simulink model "Simscape_Benchmark_SIM1"  (R2021a)
settings: Solver=ode45  StartTime=0.0  StopTime=PHASE.Ttotal  FixedStep=Benchmark.Sim.Tint  RelTol=1e-5  AbsTol=1e-6
undefined symbols (not defined in the file): Actuators, Analysis, antisym, Benchmark, Bus, Disturbance, FSM, IntialCond, ISOL, K_Coarse_disc_t, Kslew_opt_disc_zoh, Model, MPS, PAYLOAD, PHASE, PMA, RWIsol, RWS, SA, Sensors, Slew, slosh, thr, X, Y, Z
libraries: sm_lib x215, nesl_utility x148, simulink x65, cstblocks x36, sharedtransform x4, vrlib x3, RCTblocks x1
(part 9 of 9)

== system Simscape_Benchmark_SIM1/Dynamical system/WEMS + Reaction wheels/RW saturation and friction model/Saturations + friction model + friction spikes/Spike generation RW2 ==
  note: The condition above triggers the calculation of the spike level and the repetition time.
      | While the time_counter < Rep_time the trigger is not activated. As soon as the condition is met. The logical operator {>} activates the trigger_spike subsystem and resets the counter.
  note: maybe there's a better way to round up numbers to a certain decimal in simulink but that works fine for now
  note: The function counts how many times the {>} is activated. The output values is also used in the selection of the first repetition time since this is not initialized with trigger_spike.
  note: This part is done to avoid having a first spike always at t=t_duration of spike (which is 20 sec in this case)...so we have a trigger that for the first time (when the subsystem that computes the spike repetition time has still not been triggered) choose the time of the first initial spike.... the other time will be the t_duration that sums yp with the spike repetition time
  Constant16 : Constant  Value=RWS.spike.duration
  Constant17 : Constant  Value=0  SampleTime=Model.ACS_sampling.Ts
  Constant18 : Constant  Value=RWS.spike.repetition.w2_Initialization  SampleTime=Inf
  Constant4 : Constant  Value=0  SampleTime=Model.ACS_sampling.Ts
  Couter with reset function given by a condition : Subsystem
  Gain4 : Gain  Gain=10
  Gain5 : Gain  Gain=1/10
  Memory{12..15} (4 alike) : Memory
  Relational Operator3 : RelationalOperator  Operator=>  OutDataTypeStr=boolean  RndMeth=Simplest
  Round2 : Rounding  Operator=round
  Scope{5,15,20..22} (5 alike) : Scope
  Scope23 : Scope  NumInputPorts=3
  Set_spike_duration : MATLAB Function  TreatAsAtomicUnit=on
  Sum2 : Sum  Inputs=|++
  Sum8 : Sum  Inputs=|++
  Switch3 : Switch  Criteria=u2 > Threshold  Threshold=RWS.spike.duration/Model.ACS_sampling.Ts
  Switch7 : Switch  Criteria=u2 > Threshold  Threshold=1
  Trigger_spike : Subsystem  TreatAsAtomicUnit=on
  Triggered_spikes_counter : Subsystem  TreatAsAtomicUnit=on
  Out1 : Outport
  wires:
  Constant16/1 -> Switch7/1
  Sum8/1 -> Relational Operator3/2, Scope20/1
  Gain5/1 -> Switch7/3
  Set_spike_duration/1(y) -> Switch3/2, Memory15/1
  Relational Operator3/1 -> Scope23/2, Triggered_spikes_counter/Trigger, Couter with reset function given by a condition/1(In1), Trigger_spike/Trigger
  Constant18/1 -> Gain4/1
  Sum2/1 -> Set_spike_duration/3(counter)
  Constant4/1 -> Sum2/1
  Round2/1 -> Gain5/1
  Memory12/1 -> Set_spike_duration/2(uk_1)
  Memory13/1 -> Sum8/1
  Trigger_spike/1(Spike_level) -> Set_spike_duration/1(uk), Switch3/3, Memory12/1, Scope5/1, Scope23/1
  Memory14/1 -> Sum8/2
  Trigger_spike/2(Rep_time) -> Memory13/1
  Switch3/1 -> Out1/1, Scope21/1  "Spike(t)"
  Constant17/1 -> Switch3/1
  Memory15/1 -> Sum2/2
  Triggered_spikes_counter/1(Out1) -> Scope15/1, Switch7/2
  Gain4/1 -> Round2/1
  Couter with reset function given by a condition/1(Time_counter) -> Relational Operator3/1, Scope23/3
  Switch7/1 -> Scope22/1, Memory14/1

== system Simscape_Benchmark_SIM1/Dynamical system/WEMS + Reaction wheels/RW saturation and friction model/Saturations + friction model + friction spikes/Spike generation RW3 ==
  note: The condition above triggers the calculation of the spike level and the repetition time.
      | While the time_counter < Rep_time the trigger is not activated. As soon as the condition is met. The logical operator {>} activates the trigger_spike subsystem and resets the counter.
  note: maybe there's a better way to round up numbers to a certain decimal in simulink but that works fine for now
  note: The function counts how many times the {>} is activated. The output values is also used in the selection of the first repetition time since this is not initialized with trigger_spike.
  note: This part is done to avoid having a first spike always at t=t_duration of spike (which is 20 sec in this case)...so we have a trigger that for the first time (when the subsystem that computes the spike repetition time has still not been triggered) choose the time of the first initial spike.... the other time will be the t_duration that sums yp with the spike repetition time
  Constant16 : Constant  Value=RWS.spike.duration
  Constant17 : Constant  Value=0  SampleTime=Model.ACS_sampling.Ts
  Constant18 : Constant  Value=RWS.spike.repetition.w3_Initialization  SampleTime=Inf
  Constant4 : Constant  Value=0  SampleTime=Model.ACS_sampling.Ts
  Couter with reset function given by a condition : Subsystem
  Gain4 : Gain  Gain=10
  Gain5 : Gain  Gain=1/10
  Memory{12..15} (4 alike) : Memory
  Relational Operator3 : RelationalOperator  Operator=>  OutDataTypeStr=boolean  RndMeth=Simplest
  Round2 : Rounding  Operator=round
  Scope{5,15,20..22} (5 alike) : Scope
  Scope23 : Scope  NumInputPorts=3
  Set_spike_duration : MATLAB Function  TreatAsAtomicUnit=on
  Sum2 : Sum  Inputs=|++
  Sum8 : Sum  Inputs=|++
  Switch3 : Switch  Criteria=u2 > Threshold  Threshold=RWS.spike.duration/Model.ACS_sampling.Ts
  Switch7 : Switch  Criteria=u2 > Threshold  Threshold=1
  Trigger_spike : Subsystem  TreatAsAtomicUnit=on
  Triggered_spikes_counter : Subsystem  TreatAsAtomicUnit=on
  Out1 : Outport
  wires:
  Constant16/1 -> Switch7/1
  Sum8/1 -> Relational Operator3/2, Scope20/1
  Gain5/1 -> Switch7/3
  Set_spike_duration/1(y) -> Switch3/2, Memory15/1
  Relational Operator3/1 -> Scope23/2, Triggered_spikes_counter/Trigger, Couter with reset function given by a condition/1(In1), Trigger_spike/Trigger
  Constant18/1 -> Gain4/1
  Sum2/1 -> Set_spike_duration/3(counter)
  Constant4/1 -> Sum2/1
  Round2/1 -> Gain5/1
  Memory12/1 -> Set_spike_duration/2(uk_1)
  Memory13/1 -> Sum8/1
  Trigger_spike/1(Spike_level) -> Set_spike_duration/1(uk), Switch3/3, Memory12/1, Scope5/1, Scope23/1
  Memory14/1 -> Sum8/2
  Trigger_spike/2(Rep_time) -> Memory13/1
  Switch3/1 -> Out1/1, Scope21/1  "Spike(t)"
  Constant17/1 -> Switch3/1
  Memory15/1 -> Sum2/2
  Triggered_spikes_counter/1(Out1) -> Scope15/1, Switch7/2
  Gain4/1 -> Round2/1
  Couter with reset function given by a condition/1(Time_counter) -> Relational Operator3/1, Scope23/3
  Switch7/1 -> Scope22/1, Memory14/1

== system Simscape_Benchmark_SIM1/Dynamical system/WEMS + Reaction wheels/RW saturation and friction model/Saturations + friction model + friction spikes/Spike generation RW4 ==
  note: The condition above triggers the calculation of the spike level and the repetition time.
      | While the time_counter < Rep_time the trigger is not activated. As soon as the condition is met. The logical operator {>} activates the trigger_spike subsystem and resets the counter.
  note: maybe there's a better way to round up numbers to a certain decimal in simulink but that works fine for now
  note: The function counts how many times the {>} is activated. The output values is also used in the selection of the first repetition time since this is not initialized with trigger_spike.
  note: This part is done to avoid having a first spike always at t=t_duration of spike (which is 20 sec in this case)...so we have a trigger that for the first time (when the subsystem that computes the spike repetition time has still not been triggered) choose the time of the first initial spike.... the other time will be the t_duration that sums yp with the spike repetition time
  Constant16 : Constant  Value=RWS.spike.duration
  Constant17 : Constant  Value=0  SampleTime=Model.ACS_sampling.Ts
  Constant18 : Constant  Value=RWS.spike.repetition.w4_Initialization  SampleTime=Inf
  Constant4 : Constant  Value=0  SampleTime=Model.ACS_sampling.Ts
  Couter with reset function given by a condition : Subsystem
  Gain4 : Gain  Gain=10
  Gain5 : Gain  Gain=1/10
  Memory{12..15} (4 alike) : Memory
  Relational Operator3 : RelationalOperator  Operator=>  OutDataTypeStr=boolean  RndMeth=Simplest
  Round2 : Rounding  Operator=round
  Scope{5,15,20..22} (5 alike) : Scope
  Scope23 : Scope  NumInputPorts=3
  Set_spike_duration : MATLAB Function  TreatAsAtomicUnit=on
  Sum2 : Sum  Inputs=|++
  Sum8 : Sum  Inputs=|++
  Switch3 : Switch  Criteria=u2 > Threshold  Threshold=RWS.spike.duration/Model.ACS_sampling.Ts
  Switch7 : Switch  Criteria=u2 > Threshold  Threshold=1
  Trigger_spike : Subsystem  TreatAsAtomicUnit=on
  Triggered_spikes_counter : Subsystem  TreatAsAtomicUnit=on
  Out1 : Outport
  wires:
  Constant16/1 -> Switch7/1
  Sum8/1 -> Relational Operator3/2, Scope20/1
  Gain5/1 -> Switch7/3
  Set_spike_duration/1(y) -> Switch3/2, Memory15/1
  Relational Operator3/1 -> Scope23/2, Triggered_spikes_counter/Trigger, Couter with reset function given by a condition/1(In1), Trigger_spike/Trigger
  Constant18/1 -> Gain4/1
  Sum2/1 -> Set_spike_duration/3(counter)
  Constant4/1 -> Sum2/1
  Round2/1 -> Gain5/1
  Memory12/1 -> Set_spike_duration/2(uk_1)
  Memory13/1 -> Sum8/1
  Trigger_spike/1(Spike_level) -> Set_spike_duration/1(uk), Switch3/3, Memory12/1, Scope5/1, Scope23/1
  Memory14/1 -> Sum8/2
  Trigger_spike/2(Rep_time) -> Memory13/1
  Switch3/1 -> Out1/1, Scope21/1  "Spike(t)"
  Constant17/1 -> Switch3/1
  Memory15/1 -> Sum2/2
  Triggered_spikes_counter/1(Out1) -> Scope15/1, Switch7/2
  Gain4/1 -> Round2/1
  Couter with reset function given by a condition/1(Time_counter) -> Relational Operator3/1, Scope23/3
  Switch7/1 -> Scope22/1, Memory14/1

== system Simscape_Benchmark_SIM1/Dynamical system/WEMS + Reaction wheels/RW saturation and friction model/Saturations +  friction model/RW friction model/Friction model (torque) ==
  rw_speed (rad/s) : Inport
  motor cmd trq (Nm) : Inport  Port=2
  Computation of the sign of rw_speed : Subsystem
  Friction torque calculation : Subsystem
  Sum : Sum  Inputs=+++  SaturateOnIntegerOverflow=on
  Sum1 : Sum  SaturateOnIntegerOverflow=on
  Torque_total : Outport  VectorParamsAs1DForOutWhenUnconnected=off
  Torque_friction : Outport  Port=2  VectorParamsAs1DForOutWhenUnconnected=off
  wires:
  rw_speed (rad/s)/1 -> Computation of the sign of rw_speed/1(rw_speed), Friction torque calculation/1(rw_speed)
  Computation of the sign of rw_speed/1(sign_rw_speed) -> Friction torque calculation/2(sign_rw_speed)
  Friction torque calculation/2(Torque_stiction) -> Sum/2
  Friction torque calculation/1(Torque_Coulomb) -> Sum/1
  Sum1/1 -> Torque_total/1
  Friction torque calculation/3(Torque_viscous) -> Sum/3
  Sum/1 -> Torque_friction/1, Sum1/1
  motor cmd trq (Nm)/1 -> Computation of the sign of rw_speed/2(Torque_motor), Sum1/2

== system Simscape_Benchmark_SIM1/Dynamical system/WEMS + Reaction wheels/RW saturation and friction model/Saturations + friction model + friction spikes/RW friction model/Friction model (torque)1 ==
  rw_speed (rad/s) : Inport
  motor cmd trq (Nm) : Inport  Port=2
  Computation of the sign of rw_speed : Subsystem
  Friction torque calculation : Subsystem
  Sum : Sum  Inputs=+++  SaturateOnIntegerOverflow=on
  Sum1 : Sum  SaturateOnIntegerOverflow=on
  Torque_total : Outport  VectorParamsAs1DForOutWhenUnconnected=off
  Torque_friction : Outport  Port=2  VectorParamsAs1DForOutWhenUnconnected=off
  sign_omega : Outport  Port=3
  wires:
  rw_speed (rad/s)/1 -> Computation of the sign of rw_speed/1(rw_speed), Friction torque calculation/1(rw_speed)
  Friction torque calculation/2(Torque_stiction) -> Sum/2
  Friction torque calculation/1(Torque_Coulomb) -> Sum/1
  Sum1/1 -> Torque_total/1
  Friction torque calculation/3(Torque_viscous) -> Sum/3
  Sum/1 -> Torque_friction/1, Sum1/1
  motor cmd trq (Nm)/1 -> Computation of the sign of rw_speed/2(Torque_motor), Sum1/2
  Computation of the sign of rw_speed/1(sign_rw_speed) -> sign_omega/1, Friction torque calculation/2(sign_rw_speed)

== system Simscape_Benchmark_SIM1/Dynamical system/WEMS + Reaction wheels/RW saturation and friction model/Saturations + friction model + friction spikes/Spike generation RW1/Couter with reset function given by a condition ==
  note: When the IF condition of the switch is met the counter gets reset at zero
  In1 : Inport
  Constant10 : Constant  SampleTime=Model.ACS_sampling.Ts
  Constant12 : Constant  Value=0  SampleTime=Model.ACS_sampling.Ts
  Delay : Delay  DelayLength=1  SampleTime=Model.ACS_sampling.Ts
  Memory17 : Memory  InheritSampleTime=on
  Scope18 : Scope
  Sum7 : Sum  Inputs=|++
  Switch6 : Switch  Criteria=u2 > Threshold
  Ts : Gain  Gain=Model.ACS_sampling.Ts
  Time_counter : Outport
  wires:
  Sum7/1 -> Switch6/3
  Constant10/1 -> Ts/1
  Ts/1 -> Sum7/1
  Constant12/1 -> Switch6/1
  Switch6/1 -> Delay/1, Time_counter/1, Scope18/1
  In1/1 -> Memory17/1
  Memory17/1 -> Switch6/2
  Delay/1 -> Sum7/2

== system Simscape_Benchmark_SIM1/Dynamical system/WEMS + Reaction wheels/RW saturation and friction model/Saturations + friction model + friction spikes/Spike generation RW1/Trigger_spike ==
  note: way to round up at first decimal term
  Trigger : TriggerPort  VariantControl=Variant
  Constant : Constant  Value=RWS.spike.level.bias
  Constant1 : Constant  Value=RWS.spike.repetition.bias
  Gain : Gain  Gain=10
  Gain1 : Gain  Gain=1/10
  Gain2 : Gain  Gain=RWS.spike.level.scaling
  Gain3 : Gain  Gain=1/RWS.spike.level.rate
  Gain4 : Gain  Gain=1/RWS.spike.repetition.rate
  Gain5 : Gain  Gain=RWS.spike.mN2N
  Log : Math  Operator=log  SaturateOnIntegerOverflow=on
  Log2 : Math  Operator=log  SaturateOnIntegerOverflow=on
  Product : Product
  Round : Rounding  Operator=round
  Scope : Scope
  Sum : Sum  Inputs=-+
  Sum1 : Sum  Inputs=-+
  Uniform Random Number : UniformRandomNumber  Minimum=0  Seed=RWS.spike.w1seed(1)
  Uniform Random Number1 : UniformRandomNumber  Minimum=0  Seed=RWS.spike.w1seed(2)
  Uniform Random Number2 : UniformRandomNumber  Minimum=0  Seed=RWS.spike.w1seed(3)
  Spike_level : Outport
  Rep_time : Outport  Port=2
  wires:
  Gain2/1 -> Spike_level/1
  Sum1/1 -> Gain/1
  Gain1/1 -> Rep_time/1
  Gain/1 -> Round/1
  Round/1 -> Gain1/1
  Uniform Random Number/1 -> Product/1
  Uniform Random Number1/1 -> Product/2
  Constant/1 -> Sum/2
  Gain5/1 -> Gain2/1
  Product/1 -> Log/1
  Log/1 -> Gain3/1
  Gain3/1 -> Scope/1, Sum/1
  Gain4/1 -> Sum1/1
  Uniform Random Number2/1 -> Log2/1
  Constant1/1 -> Sum1/2
  Log2/1 -> Gain4/1
  Sum/1 -> Gain5/1

== system Simscape_Benchmark_SIM1/Dynamical system/WEMS + Reaction wheels/RW saturation and friction model/Saturations + friction model + friction spikes/Spike generation RW1/Triggered_spikes_counter ==
  Trigger : TriggerPort  VariantControl=Variant
  Constant12 : Constant  Value=0
  Increment Stored Integer2 : simulink/Additional Math & Discrete/Additional Math: Increment - Decrement/Increment Stored Integer
  Sum8 : Sum
  Unit Delay1 : UnitDelay  SampleTime=-1  HasFrameUpgradeWarning=on
  Out1 : Outport
  wires:
  Constant12/1 -> Sum8/2
  Sum8/1 -> Increment Stored Integer2/1
  Unit Delay1/1 -> Sum8/1
  Increment Stored Integer2/1 -> Unit Delay1/1, Out1/1

== system Simscape_Benchmark_SIM1/Dynamical system/WEMS + Reaction wheels/RW saturation and friction model/Saturations + friction model + friction spikes/Spike generation RW2/Couter with reset function given by a condition ==
  note: When the IF condition of the switch is met the counter gets reset at zero
  In1 : Inport
  Constant10 : Constant  SampleTime=Model.ACS_sampling.Ts
  Constant12 : Constant  Value=0  SampleTime=Model.ACS_sampling.Ts
  Delay : Delay  DelayLength=1  SampleTime=Model.ACS_sampling.Ts
  Memory17 : Memory
  Scope18 : Scope
  Sum7 : Sum  Inputs=|++
  Switch6 : Switch  Criteria=u2 > Threshold
  Ts : Gain  Gain=Model.ACS_sampling.Ts
  Time_counter : Outport
  wires:
  Sum7/1 -> Switch6/3
  Constant10/1 -> Ts/1
  Ts/1 -> Sum7/1
  Constant12/1 -> Switch6/1
  Switch6/1 -> Delay/1, Time_counter/1, Scope18/1
  In1/1 -> Memory17/1
  Memory17/1 -> Switch6/2
  Delay/1 -> Sum7/2

== system Simscape_Benchmark_SIM1/Dynamical system/WEMS + Reaction wheels/RW saturation and friction model/Saturations + friction model + friction spikes/Spike generation RW2/Trigger_spike ==
  note: way to round up at first decimal term
  Trigger : TriggerPort  VariantControl=Variant
  Constant : Constant  Value=RWS.spike.level.bias
  Constant1 : Constant  Value=RWS.spike.repetition.bias
  Gain : Gain  Gain=10
  Gain1 : Gain  Gain=1/10
  Gain2 : Gain  Gain=RWS.spike.level.scaling
  Gain3 : Gain  Gain=1/RWS.spike.level.rate
  Gain4 : Gain  Gain=1/RWS.spike.repetition.rate
  Gain5 : Gain  Gain=RWS.spike.mN2N
  Log : Math  Operator=log  SaturateOnIntegerOverflow=on
  Log2 : Math  Operator=log  SaturateOnIntegerOverflow=on
  Product : Product
  Round : Rounding  Operator=round
  Scope : Scope
  Sum : Sum  Inputs=-+
  Sum1 : Sum  Inputs=-+
  Uniform Random Number : UniformRandomNumber  Minimum=0  Seed=RWS.spike.w2seed(1)
  Uniform Random Number1 : UniformRandomNumber  Minimum=0  Seed=RWS.spike.w2seed(2)
  Uniform Random Number2 : UniformRandomNumber  Minimum=0  Seed=RWS.spike.w2seed(3)
  Spike_level : Outport
  Rep_time : Outport  Port=2
  wires:
  Gain2/1 -> Spike_level/1
  Sum1/1 -> Gain/1
  Gain1/1 -> Rep_time/1
  Gain/1 -> Round/1
  Round/1 -> Gain1/1
  Uniform Random Number/1 -> Product/1
  Uniform Random Number1/1 -> Product/2
  Constant/1 -> Sum/2
  Gain5/1 -> Gain2/1
  Product/1 -> Log/1
  Log/1 -> Gain3/1
  Gain3/1 -> Scope/1, Sum/1
  Gain4/1 -> Sum1/1
  Uniform Random Number2/1 -> Log2/1
  Constant1/1 -> Sum1/2
  Log2/1 -> Gain4/1
  Sum/1 -> Gain5/1

== system Simscape_Benchmark_SIM1/Dynamical system/WEMS + Reaction wheels/RW saturation and friction model/Saturations + friction model + friction spikes/Spike generation RW2/Triggered_spikes_counter ==
  Trigger : TriggerPort  VariantControl=Variant
  Constant12 : Constant  Value=0
  Increment Stored Integer2 : simulink/Additional Math & Discrete/Additional Math: Increment - Decrement/Increment Stored Integer
  Sum8 : Sum
  Unit Delay1 : UnitDelay  SampleTime=-1  HasFrameUpgradeWarning=on
  Out1 : Outport
  wires:
  Constant12/1 -> Sum8/2
  Sum8/1 -> Increment Stored Integer2/1
  Unit Delay1/1 -> Sum8/1
  Increment Stored Integer2/1 -> Unit Delay1/1, Out1/1

== system Simscape_Benchmark_SIM1/Dynamical system/WEMS + Reaction wheels/RW saturation and friction model/Saturations + friction model + friction spikes/Spike generation RW3/Couter with reset function given by a condition ==
  note: When the IF condition of the switch is met the counter gets reset at zero
  In1 : Inport
  Constant10 : Constant  SampleTime=Model.ACS_sampling.Ts
  Constant12 : Constant  Value=0  SampleTime=Model.ACS_sampling.Ts
  Delay : Delay  DelayLength=1  SampleTime=Model.ACS_sampling.Ts
  Memory17 : Memory
  Scope18 : Scope
  Sum7 : Sum  Inputs=|++
  Switch6 : Switch  Criteria=u2 > Threshold
  Ts : Gain  Gain=Model.ACS_sampling.Ts
  Time_counter : Outport
  wires:
  Sum7/1 -> Switch6/3
  Constant10/1 -> Ts/1
  Ts/1 -> Sum7/1
  Constant12/1 -> Switch6/1
  Switch6/1 -> Delay/1, Time_counter/1, Scope18/1
  In1/1 -> Memory17/1
  Memory17/1 -> Switch6/2
  Delay/1 -> Sum7/2

== system Simscape_Benchmark_SIM1/Dynamical system/WEMS + Reaction wheels/RW saturation and friction model/Saturations + friction model + friction spikes/Spike generation RW3/Trigger_spike ==
  note: way to round up at first decimal term
  Trigger : TriggerPort  VariantControl=Variant
  Constant : Constant  Value=RWS.spike.level.bias
  Constant1 : Constant  Value=RWS.spike.repetition.bias
  Gain : Gain  Gain=10
  Gain1 : Gain  Gain=1/10
  Gain2 : Gain  Gain=RWS.spike.level.scaling
  Gain3 : Gain  Gain=1/RWS.spike.level.rate
  Gain4 : Gain  Gain=1/RWS.spike.repetition.rate
  Gain5 : Gain  Gain=RWS.spike.mN2N
  Log : Math  Operator=log  SaturateOnIntegerOverflow=on
  Log2 : Math  Operator=log  SaturateOnIntegerOverflow=on
  Product : Product
  Round : Rounding  Operator=round
  Scope : Scope
  Sum : Sum  Inputs=-+
  Sum1 : Sum  Inputs=-+
  Uniform Random Number : UniformRandomNumber  Minimum=0  Seed=RWS.spike.w3seed(1)
  Uniform Random Number1 : UniformRandomNumber  Minimum=0  Seed=RWS.spike.w3seed(2)
  Uniform Random Number2 : UniformRandomNumber  Minimum=0  Seed=RWS.spike.w3seed(3)
  Spike_level : Outport
  Rep_time : Outport  Port=2
  wires:
  Gain2/1 -> Spike_level/1
  Sum1/1 -> Gain/1
  Gain1/1 -> Rep_time/1
  Gain/1 -> Round/1
  Round/1 -> Gain1/1
  Uniform Random Number/1 -> Product/1
  Uniform Random Number1/1 -> Product/2
  Constant/1 -> Sum/2
  Gain5/1 -> Gain2/1
  Product/1 -> Log/1
  Log/1 -> Gain3/1
  Gain3/1 -> Scope/1, Sum/1
  Gain4/1 -> Sum1/1
  Uniform Random Number2/1 -> Log2/1
  Constant1/1 -> Sum1/2
  Log2/1 -> Gain4/1
  Sum/1 -> Gain5/1

== system Simscape_Benchmark_SIM1/Dynamical system/WEMS + Reaction wheels/RW saturation and friction model/Saturations + friction model + friction spikes/Spike generation RW3/Triggered_spikes_counter ==
  Trigger : TriggerPort  VariantControl=Variant
  Constant12 : Constant  Value=0
  Increment Stored Integer2 : simulink/Additional Math & Discrete/Additional Math: Increment - Decrement/Increment Stored Integer
  Sum8 : Sum
  Unit Delay1 : UnitDelay  SampleTime=-1  HasFrameUpgradeWarning=on
  Out1 : Outport
  wires:
  Constant12/1 -> Sum8/2
  Sum8/1 -> Increment Stored Integer2/1
  Unit Delay1/1 -> Sum8/1
  Increment Stored Integer2/1 -> Unit Delay1/1, Out1/1

== system Simscape_Benchmark_SIM1/Dynamical system/WEMS + Reaction wheels/RW saturation and friction model/Saturations + friction model + friction spikes/Spike generation RW4/Couter with reset function given by a condition ==
  note: When the IF condition of the switch is met the counter gets reset at zero
  In1 : Inport
  Constant10 : Constant  SampleTime=Model.ACS_sampling.Ts
  Constant12 : Constant  Value=0  SampleTime=Model.ACS_sampling.Ts
  Delay : Delay  DelayLength=1  SampleTime=Model.ACS_sampling.Ts
  Memory17 : Memory
  Scope18 : Scope
  Sum7 : Sum  Inputs=|++
  Switch6 : Switch  Criteria=u2 > Threshold
  Ts : Gain  Gain=Model.ACS_sampling.Ts
  Time_counter : Outport
  wires:
  Sum7/1 -> Switch6/3
  Constant10/1 -> Ts/1
  Ts/1 -> Sum7/1
  Constant12/1 -> Switch6/1
  Switch6/1 -> Delay/1, Time_counter/1, Scope18/1
  In1/1 -> Memory17/1
  Memory17/1 -> Switch6/2
  Delay/1 -> Sum7/2

== system Simscape_Benchmark_SIM1/Dynamical system/WEMS + Reaction wheels/RW saturation and friction model/Saturations + friction model + friction spikes/Spike generation RW4/Trigger_spike ==
  note: way to round up at first decimal term
  Trigger : TriggerPort  VariantControl=Variant
  Constant : Constant  Value=RWS.spike.level.bias
  Constant1 : Constant  Value=RWS.spike.repetition.bias
  Gain : Gain  Gain=10
  Gain1 : Gain  Gain=1/10
  Gain2 : Gain  Gain=RWS.spike.level.scaling
  Gain3 : Gain  Gain=1/RWS.spike.level.rate
  Gain4 : Gain  Gain=1/RWS.spike.repetition.rate
  Gain5 : Gain  Gain=RWS.spike.mN2N
  Log : Math  Operator=log  SaturateOnIntegerOverflow=on
  Log2 : Math  Operator=log  SaturateOnIntegerOverflow=on
  Product : Product
  Round : Rounding  Operator=round
  Scope : Scope
  Sum : Sum  Inputs=-+
  Sum1 : Sum  Inputs=-+
  Uniform Random Number : UniformRandomNumber  Minimum=0  Seed=RWS.spike.w4seed(1)
  Uniform Random Number1 : UniformRandomNumber  Minimum=0  Seed=RWS.spike.w4seed(2)
  Uniform Random Number2 : UniformRandomNumber  Minimum=0  Seed=RWS.spike.w4seed(3)
  Spike_level : Outport
  Rep_time : Outport  Port=2
  wires:
  Gain2/1 -> Spike_level/1
  Sum1/1 -> Gain/1
  Gain1/1 -> Rep_time/1
  Gain/1 -> Round/1
  Round/1 -> Gain1/1
  Uniform Random Number/1 -> Product/1
  Uniform Random Number1/1 -> Product/2
  Constant/1 -> Sum/2
  Gain5/1 -> Gain2/1
  Product/1 -> Log/1
  Log/1 -> Gain3/1
  Gain3/1 -> Scope/1, Sum/1
  Gain4/1 -> Sum1/1
  Uniform Random Number2/1 -> Log2/1
  Constant1/1 -> Sum1/2
  Log2/1 -> Gain4/1
  Sum/1 -> Gain5/1

== system Simscape_Benchmark_SIM1/Dynamical system/WEMS + Reaction wheels/RW saturation and friction model/Saturations + friction model + friction spikes/Spike generation RW4/Triggered_spikes_counter ==
  Trigger : TriggerPort  VariantControl=Variant
  Constant12 : Constant  Value=0
  Increment Stored Integer2 : simulink/Additional Math & Discrete/Additional Math: Increment - Decrement/Increment Stored Integer
  Sum8 : Sum
  Unit Delay1 : UnitDelay  SampleTime=-1  HasFrameUpgradeWarning=on
  Out1 : Outport
  wires:
  Constant12/1 -> Sum8/2
  Sum8/1 -> Increment Stored Integer2/1
  Unit Delay1/1 -> Sum8/1
  Increment Stored Integer2/1 -> Unit Delay1/1, Out1/1

== system Simscape_Benchmark_SIM1/Dynamical system/WEMS + Reaction wheels/RW saturation and friction model/Saturations +  friction model/RW friction model/Friction model (torque)/Computation of the sign of rw_speed ==
  note: IF [rw_speed| <= eps AND |Torque_motor|>eps then:
      | sign( rw_speed )=Torque_motor/|Torque_motor|
      |
      | IF [ rw_speed | <= eps and | Torque_motor |<= eps then sign( rw_speed )=0 so zero friction
  note: IF |rw_speed|>eps (tolerance given in input):
      | Then sign(rw_speed)=rw_speed/|rw_speed|
  rw_speed : Inport
  Torque_motor : Inport  Port=2
  Abs2 : Abs  SaturateOnIntegerOverflow=on
  Abs3 : Abs  SaturateOnIntegerOverflow=on
  Add : Sum  Inputs=+++
  Constant{2..5} (4 alike) : Constant  Value=zeros(1,length(RWS.eps))
  Logical Operator : Logic  AllPortsSameDT=off  OutDataTypeStr=boolean
  Logical Operator1 : Logic  AllPortsSameDT=off  OutDataTypeStr=boolean
  Relational Operator : RelationalOperator  Operator=>  OutDataTypeStr=boolean  ZeroCross=off  RndMeth=Nearest
  Relational Operator1 : RelationalOperator  Operator=<=  OutDataTypeStr=boolean  RndMeth=Nearest
  Relational Operator2 : RelationalOperator  Operator=>  OutDataTypeStr=boolean  ZeroCross=off  RndMeth=Nearest
  Relational Operator3 : RelationalOperator  Operator=<=  OutDataTypeStr=boolean  ZeroCross=off  RndMeth=Nearest
  Sign2 : Signum  ZeroCross=off
  Sign4 : Signum
  Switch1 : Switch  Criteria=u2 > Threshold  ZeroCross=off
  Switch2 : Switch  Criteria=u2 > Threshold  ZeroCross=off
  Switch3 : Switch  Criteria=u2 > Threshold  ZeroCross=off
  rw.eps1 : Constant  Value=RWS.eps
  sign_rw_speed : Outport  VectorParamsAs1DForOutWhenUnconnected=off
  wires:
  Logical Operator1/1 -> Switch3/2
  Logical Operator/1 -> Switch2/2
  Relational Operator3/1 -> Logical Operator1/2
  Relational Operator2/1 -> Logical Operator/2
  Abs3/1 -> Relational Operator3/1, Relational Operator2/1
  Relational Operator1/1 -> Logical Operator1/1, Logical Operator/1
  rw.eps1/1 -> Relational Operator/2, Relational Operator1/2, Relational Operator3/2, Relational Operator2/2
  Abs2/1 -> Relational Operator1/1, Relational Operator/1
  rw_speed/1 -> Sign4/1, Abs2/1
  Switch2/1 -> Add/2
  Constant5/1 -> Switch3/1
  Constant3/1 -> Switch2/3
  Sign4/1 -> Switch1/1
  Relational Operator/1 -> Switch1/2
  Switch1/1 -> Add/1
  Constant4/1 -> Switch3/3
  Constant2/1 -> Switch1/3
  Switch3/1 -> Add/3
  Sign2/1 -> Switch2/1
  Add/1 -> sign_rw_speed/1
  Torque_motor/1 -> Sign2/1, Abs3/1

== system Simscape_Benchmark_SIM1/Dynamical system/WEMS + Reaction wheels/RW saturation and friction model/Saturations +  friction model/RW friction model/Friction model (torque)/Friction torque calculation ==
  note: IF |rw_speed|<=RWS.w_threshold then:
      |
      | Torque_stiction=-k_stiction*sign(rw_speed)
      |
      | otherwise Torque_stiction=0
  note: IF |rw_speed|>RWS.w_threshold then:
      |
      | Torque_Coulomb=-k_Coulomb*sign(rw_speed)
      |
      | otherwise Torque_Coulomb=0
  note: Torque_viscous=-k_viscous* rw_speed
  rw_speed : Inport
  sign_rw_speed : Inport  Port=2
  Abs : Abs  SaturateOnIntegerOverflow=on
  Gain : Gain  Gain=-1  SaturateOnIntegerOverflow=on  OutDataTypeStr=Inherit: Same as input  ParamDataTypeStr=Inherit: Same as input
  Gain1 : Gain  Gain=-1  SaturateOnIntegerOverflow=on  OutDataTypeStr=Inherit: Same as input  ParamDataTypeStr=Inherit: Same as input
  Gain2 : Gain  Gain=-1  SaturateOnIntegerOverflow=on  OutDataTypeStr=Inherit: Same as input  ParamDataTypeStr=Inherit: Same as input
  Switch : Switch  Threshold=RWS.w_threshold  ZeroCross=off  SaturateOnIntegerOverflow=on
  Switch2 : Switch  Threshold=RWS.w_threshold  ZeroCross=off  SaturateOnIntegerOverflow=on
  Torque_Coulomb=0 : Constant  Value=0
  Torque_stiction=0 : Constant  Value=0
  k_Coulomb : Gain  Gain=RWS.k_coulomb  SaturateOnIntegerOverflow=on  OutDataTypeStr=Inherit: Same as input  ParamDataTypeStr=Inherit: Same as input
  k_stiction : Gain  Gain=RWS.k_stiction  SaturateOnIntegerOverflow=on  OutDataTypeStr=Inherit: Same as input  ParamDataTypeStr=Inherit: Same as input
  k_viscous : Gain  Gain=RWS.k_viscous  SaturateOnIntegerOverflow=on  OutDataTypeStr=Inherit: Same as input  ParamDataTypeStr=Inherit: Same as input
  Torque_Coulomb : Outport  VectorParamsAs1DForOutWhenUnconnected=off
  Torque_stiction : Outport  Port=2  VectorParamsAs1DForOutWhenUnconnected=off
  Torque_viscous : Outport  Port=3  VectorParamsAs1DForOutWhenUnconnected=off
  wires:
  k_viscous/1 -> Torque_viscous/1
  Gain2/1 -> k_viscous/1
  Torque_stiction=0/1 -> Switch2/1
  k_stiction/1 -> Switch2/3
  Torque_Coulomb=0/1 -> Switch/3
  k_Coulomb/1 -> Switch/1
  Gain1/1 -> k_stiction/1
  Gain/1 -> k_Coulomb/1
  rw_speed/1 -> Gain2/1, Abs/1
  Abs/1 -> Switch2/2, Switch/2
  sign_rw_speed/1 -> Gain1/1, Gain/1
  Switch/1 -> Torque_Coulomb/1
  Switch2/1 -> Torque_stiction/1

== system Simscape_Benchmark_SIM1/Dynamical system/WEMS + Reaction wheels/RW saturation and friction model/Saturations + friction model + friction spikes/RW friction model/Friction model (torque)1/Computation of the sign of rw_speed ==
  note: IF [rw_speed| <= eps AND |Torque_motor|>eps then:
      | sign( rw_speed )=Torque_motor/|Torque_motor|
      |
      | IF [ rw_speed | <= eps and | Torque_motor |<= eps then sign( rw_speed )=0 so zero friction
  note: IF |rw_speed|>eps (tolerance given in input):
      | Then sign(rw_speed)=rw_speed/|rw_speed|
  rw_speed : Inport
  Torque_motor : Inport  Port=2
  Abs2 : Abs  SaturateOnIntegerOverflow=on
  Abs3 : Abs  SaturateOnIntegerOverflow=on
  Add : Sum  Inputs=+++
  Constant{2..5} (4 alike) : Constant  Value=zeros(1,length(RWS.eps))
  Logical Operator : Logic  AllPortsSameDT=off  OutDataTypeStr=boolean
  Logical Operator1 : Logic  AllPortsSameDT=off  OutDataTypeStr=boolean
  Relational Operator : RelationalOperator  Operator=>  OutDataTypeStr=boolean  ZeroCross=off  RndMeth=Nearest
  Relational Operator1 : RelationalOperator  Operator=<=  OutDataTypeStr=boolean  RndMeth=Nearest
  Relational Operator2 : RelationalOperator  Operator=>  OutDataTypeStr=boolean  ZeroCross=off  RndMeth=Nearest
  Relational Operator3 : RelationalOperator  Operator=<=  OutDataTypeStr=boolean  ZeroCross=off  RndMeth=Nearest
  Sign2 : Signum  ZeroCross=off
  Sign4 : Signum
  Switch1 : Switch  Criteria=u2 > Threshold  ZeroCross=off
  Switch2 : Switch  Criteria=u2 > Threshold  ZeroCross=off
  Switch3 : Switch  Criteria=u2 > Threshold  ZeroCross=off
  rw.eps1 : Constant  Value=RWS.eps
  sign_rw_speed : Outport  VectorParamsAs1DForOutWhenUnconnected=off
  wires:
  Logical Operator1/1 -> Switch3/2
  Logical Operator/1 -> Switch2/2
  Relational Operator3/1 -> Logical Operator1/2
  Relational Operator2/1 -> Logical Operator/2
  Abs3/1 -> Relational Operator3/1, Relational Operator2/1
  Relational Operator1/1 -> Logical Operator1/1, Logical Operator/1
  rw.eps1/1 -> Relational Operator/2, Relational Operator1/2, Relational Operator3/2, Relational Operator2/2
  Abs2/1 -> Relational Operator1/1, Relational Operator/1
  rw_speed/1 -> Sign4/1, Abs2/1
  Switch2/1 -> Add/2
  Constant5/1 -> Switch3/1
  Constant3/1 -> Switch2/3
  Sign4/1 -> Switch1/1
  Relational Operator/1 -> Switch1/2
  Switch1/1 -> Add/1
  Constant4/1 -> Switch3/3
  Constant2/1 -> Switch1/3
  Switch3/1 -> Add/3
  Sign2/1 -> Switch2/1
  Add/1 -> sign_rw_speed/1
  Torque_motor/1 -> Sign2/1, Abs3/1

== system Simscape_Benchmark_SIM1/Dynamical system/WEMS + Reaction wheels/RW saturation and friction model/Saturations + friction model + friction spikes/RW friction model/Friction model (torque)1/Friction torque calculation ==
  note: IF |rw_speed|<=RWS.w_threshold then:
      |
      | Torque_stiction=-k_stiction*sign(rw_speed)
      |
      | otherwise Torque_stiction=0
  note: IF |rw_speed|>RWS.w_threshold then:
      |
      | Torque_Coulomb=-k_Coulomb*sign(rw_speed)
      |
      | otherwise Torque_Coulomb=0
  note: Torque_viscous=-k_viscous* rw_speed
  rw_speed : Inport
  sign_rw_speed : Inport  Port=2
  Abs : Abs  SaturateOnIntegerOverflow=on
  Gain : Gain  Gain=-1  SaturateOnIntegerOverflow=on  OutDataTypeStr=Inherit: Same as input  ParamDataTypeStr=Inherit: Same as input
  Gain1 : Gain  Gain=-1  SaturateOnIntegerOverflow=on  OutDataTypeStr=Inherit: Same as input  ParamDataTypeStr=Inherit: Same as input
  Gain2 : Gain  Gain=-1  SaturateOnIntegerOverflow=on  OutDataTypeStr=Inherit: Same as input  ParamDataTypeStr=Inherit: Same as input
  Switch : Switch  Threshold=RWS.w_threshold  ZeroCross=off  SaturateOnIntegerOverflow=on
  Switch2 : Switch  Threshold=RWS.w_threshold  ZeroCross=off  SaturateOnIntegerOverflow=on
  Torque_Coulomb=0 : Constant  Value=0
  Torque_stiction=0 : Constant  Value=0
  k_Coulomb : Gain  Gain=RWS.k_coulomb  SaturateOnIntegerOverflow=on  OutDataTypeStr=Inherit: Same as input  ParamDataTypeStr=Inherit: Same as input
  k_stiction : Gain  Gain=RWS.k_stiction  SaturateOnIntegerOverflow=on  OutDataTypeStr=Inherit: Same as input  ParamDataTypeStr=Inherit: Same as input
  k_viscous : Gain  Gain=RWS.k_viscous  SaturateOnIntegerOverflow=on  OutDataTypeStr=Inherit: Same as input  ParamDataTypeStr=Inherit: Same as input
  Torque_Coulomb : Outport  VectorParamsAs1DForOutWhenUnconnected=off
  Torque_stiction : Outport  Port=2  VectorParamsAs1DForOutWhenUnconnected=off
  Torque_viscous : Outport  Port=3  VectorParamsAs1DForOutWhenUnconnected=off
  wires:
  k_viscous/1 -> Torque_viscous/1
  Gain2/1 -> k_viscous/1
  Torque_stiction=0/1 -> Switch2/1
  k_stiction/1 -> Switch2/3
  Torque_Coulomb=0/1 -> Switch/3
  k_Coulomb/1 -> Switch/1
  Gain1/1 -> k_stiction/1
  Gain/1 -> k_Coulomb/1
  rw_speed/1 -> Gain2/1, Abs/1
  Abs/1 -> Switch2/2, Switch/2
  sign_rw_speed/1 -> Gain1/1, Gain/1
  Switch/1 -> Torque_Coulomb/1
  Switch2/1 -> Torque_stiction/1

== matlab function Simscape_Benchmark_SIM1/Dynamical system/RCS models/RCS (thruster model)/MATLAB Function1 ==
  data: U_cont input; u_thr input; y output; Sampling_time input; u_min input; nb_thr input; Time input; y_size input
function y = PMW_function_V2(U_cont,u_thr,Sampling_time,u_min,nb_thr,Time,y_size)

%-------------------------------------------------------------------------
% Copyright (c) ISAE-SUPAERO, All Rights Reserved.
% Paolo Iannelli, Francesco Sanfedino, Daniel Alazard (2024)
%-------------------------------------------------------------------------

% Inputs:
%   U_cont:         vecotr of the thrusts after simplex algorithm in the range
%                   [0,u_thr] - size: [1,nb_thr]
%   u_thr:          Magnitude of the thrusters [N]
%   Sampling_time:  Sampling_time [s]
%   u_min:          Computed from the MIB [N]
%   nb_thr:         Number of thrusters
%   Time:           Simulation time [s] 
%   y_size:         Initialize the vector y (zeros(thr.nb_thr,1))

eps=2e-3;

y=y_size;                           % Define the size of the output vector
K_sample=floor(Time/Sampling_time); % Time sample

%u_PWM=sign(U_cont)*u_thr;           % Vector with values of the PWM signal
u_PWM=u_thr*ones(nb_thr,1); 

% index_low: Find the thrusters that in, that time interval, cannot provide
%            the required force (since what is required is lower that the
%            specification given by the Minimum Impulse Bit)
index_low        =  find(abs(U_cont)<u_min);   

% index_value: Find the thrusters that, in that time interval, can be
%              activated and the required force is lower that the saturation 
%              level (for this it is computed the start of the pulse and its
%              duration)
index_value      =  find(abs(U_cont)>=u_min & abs(U_cont)<u_thr-eps); 

% index_saturation: Find the thrusters that, in that time interval, are
%                   activated for the full duration of the interval since
%                   the required force value is over the saturation level

index_saturation =  find(abs(U_cont)>=u_thr-eps);

% Duration of the pulse ( Vector of size:  size: [1,nb_thr])
sigma_PWM=Sampling_time*(U_cont./u_PWM);

% Delay applied to the pulse (The pulse does not begin at the start of the
% sampling period). tau_PWM=0 when we reach saturation.
tau_PWM=(Sampling_time-sigma_PWM)/2;
    
    for i=1:nb_thr
        
        if sum(i==index_low)==1 % lower than MIB = 0
            y(i)=0;
        elseif sum(i==index_saturation)==1 % saturation equal open for the full interval (there is a small activation time equal to  0.005 s)
            y(i)=u_PWM(i);  
        elseif sum(i==index_value)==1 % The pulse is centered in the interval with the delay tau_PWM
        
            if  Time-K_sample*Sampling_time-tau_PWM(i)<0 
                y(i)=0;  
            elseif Time-K_sample*Sampling_time-tau_PWM(i)>=0 & Time-K_sample*Sampling_time-tau_PWM(i)-sigma_PWM(i)<=0
                y(i)=u_PWM(i);  
            elseif Time-K_sample*Sampling_time-tau_PWM(i)-sigma_PWM(i)>0
                y(i)=0;  
            end
            
        end
    
    end

== matlab function Simscape_Benchmark_SIM1/Dynamical system/WEMS + Reaction wheels/RW saturation and friction model/Saturations + friction model + friction spikes/Spike generation RW1/Set_spike_duration ==
  data: uk input; uk_1 input; y output; counter input
function y = fcn(uk,uk_1,counter)

if uk==uk_1
y = counter+1;
else 
  y=0;
end

== matlab function Simscape_Benchmark_SIM1/Dynamical system/WEMS + Reaction wheels/RW saturation and friction model/Saturations + friction model + friction spikes/Spike generation RW2/Set_spike_duration ==
  data: uk input; uk_1 input; y output; counter input
function y = fcn(uk,uk_1,counter)

if uk==uk_1
y = counter+1;
else 
  y=0;
end

== matlab function Simscape_Benchmark_SIM1/Dynamical system/WEMS + Reaction wheels/RW saturation and friction model/Saturations + friction model + friction spikes/Spike generation RW3/Set_spike_duration ==
  data: uk input; uk_1 input; y output; counter input
function y = fcn(uk,uk_1,counter)

if uk==uk_1
y = counter+1;
else 
  y=0;
end

== matlab function Simscape_Benchmark_SIM1/Checks on pointing requirements for initiating phase transitions /Check slew APE req. ==
  data: LOS input; out output; Steady_state input; Slew_APEreq input; reference input
function out = fcn(LOS, Steady_state, Slew_APEreq, reference)

% 06/06/2024: Added addition condition (the reference signal needs to be in
% the range +-5 % of the steady state value)
if sum(abs(LOS-Steady_state)-Slew_APEreq<0)==3 & abs(reference-Steady_state)<=0.05*abs(Steady_state)
   out=1;
else
   out=0;
end

== matlab function Simscape_Benchmark_SIM1/Dynamical system/WEMS + Reaction wheels/RW saturation and friction model/Saturations + friction model + friction spikes/Spike generation RW4/Set_spike_duration ==
  data: uk input; uk_1 input; y output; counter input
function y = fcn(uk,uk_1,counter)

if uk==uk_1
y = counter+1;
else 
  y=0;
end

== matlab function Simscape_Benchmark_SIM1/Checks on pointing requirements for initiating phase transitions /Check condition for a time window (S)  ==
  data: u input; out output; sampling input; Slew_timeCheck input
function out = FUNZ(u, sampling, Slew_timeCheck)
persistent Counter_slew fix_slew
% maybe an and to deactivate it completerly

if isempty(fix_slew) 
    fix_slew=0;
end

if isempty(Counter_slew) || u==0
    Counter_slew=0;
elseif  u==1
    Counter_slew=Counter_slew+1;

end
Time_check=Counter_slew*sampling;

if Time_check>=Slew_timeCheck
    out=1;
    fix_slew=1;
else
    out=0;
end

if fix_slew==1
   out=1;
end

== matlab function Simscape_Benchmark_SIM1/Checks on pointing requirements for initiating phase transitions /Check coarse APE req. ==
  data: LOS input; out output; Steady_state input; Coarse_APEreq input; Slew_completed input
function out = fcn( LOS, Steady_state, Coarse_APEreq, Slew_completed)

if Slew_completed>0
    
        if sum(abs(LOS-Steady_state)-Coarse_APEreq<0)==3
            out=1;
        else
            out=0;
        end
else 
        
    out=0;
    
end

== matlab function Simscape_Benchmark_SIM1/Checks on pointing requirements for initiating phase transitions /Check condition for a time window (S2C) ==
  data: u input; out output; sampling input; Transition_S2CtimeCheck input; Slew_completed input; out2 output; Transition_S2CtimeCheck_reqNotMet input
function [out,out2] = FUNZ(u, sampling, Transition_S2CtimeCheck, Slew_completed, Transition_S2CtimeCheck_reqNotMet)
persistent Counter_S2C fix_transitionS2C Counter_S2C_req_NotMet

out2=1; % I have to initialize it

 if isempty(fix_transitionS2C) 
    fix_transitionS2C=0;
end
 
if isempty(Counter_S2C) || u==0
    Counter_S2C=0;
elseif  u==1
    Counter_S2C=Counter_S2C+1;
end

% This second counter starts to count as soon as the slew is completed
if isempty(Counter_S2C_req_NotMet) || Slew_completed==0
    Counter_S2C_req_NotMet=0;
elseif  Slew_completed==1
    Counter_S2C_req_NotMet=Counter_S2C_req_NotMet+1;
end
    
Time_check=Counter_S2C*sampling;
Time_check_req_NotMet=Counter_S2C_req_NotMet*sampling;

if Time_check>=Transition_S2CtimeCheck
    out=1;
    fix_transitionS2C=1;
else
    out=0;
end

% this allows tow fix the output and avoid the reactivation of a previous
% phase
if fix_transitionS2C==1 
     out=1;
     Time_check_req_NotMet=0;
     out2=1; % MEANS THAT THE REQUIREMENT IS MET
end

if Time_check_req_NotMet>=Transition_S2CtimeCheck_reqNotMet
    out=1;
    out2= 0;  % MEANS THAT THE REQUIREMENT IS not  MET
end

== matlab function Simscape_Benchmark_SIM1/Checks on pointing requirements for initiating phase transitions /Duration of Coarse ==
  data: S2C_completed input; out output; sampling input; CoarseDuration input
function out = funct_CoarseDuration(S2C_completed, sampling, CoarseDuration)
persistent Counter_CoarseDuration

    
if isempty(Counter_CoarseDuration)
    Counter_CoarseDuration=0;
elseif  S2C_completed==1
    Counter_CoarseDuration=Counter_CoarseDuration+1;

end
Time_check=Counter_CoarseDuration*sampling;

if Time_check>=CoarseDuration
    out=1;
else
    out=0;
end

== matlab function Simscape_Benchmark_SIM1/Controllers/Coarse 2 fine /Activation of fine controller ==
  data: TransitionCoarse2FineActivation input; sampling input; out output; Slope input
function out = switching_fine( TransitionCoarse2FineActivation,sampling,Slope)
persistent Counter_switching

    if isempty(Counter_switching)
    Counter_switching=0;
    elseif TransitionCoarse2FineActivation==0
    Counter_switching=0;
    elseif TransitionCoarse2FineActivation==1
    Counter_switching=Counter_switching+1;
    end
    
Time=Counter_switching*sampling;  
y=Slope*Time;

if y<1
  out=y;
else
  out=1;
end


end

== matlab function Simscape_Benchmark_SIM1/Controllers/TransitionSlew2Coarse/Slew 2 coarse switching ==
  data: TransitionCoarse2FineActivation input; sampling input; out1 output; Slope input; out2 output
function [out1,out2] = swithching_Coarse( TransitionCoarse2FineActivation,sampling,Slope)
persistent Counter_Coarse_switching

    if isempty(Counter_Coarse_switching)
    Counter_Coarse_switching=0;
    elseif TransitionCoarse2FineActivation==0
    Counter_Coarse_switching=0;
    elseif TransitionCoarse2FineActivation==1
    Counter_Coarse_switching=Counter_Coarse_switching+1;
    end
    
Time=Counter_Coarse_switching*sampling;  
y2=Slope*Time;
y1=1-Slope*Time;


if y2<1
  out1=y1;
  out2=y2;
else
  out1=0;
  out2=1;
end


end

== matlab function Simscape_Benchmark_SIM1/Checks on pointing requirements for initiating phase transitions /Check Fine APE ==
  data: LOS input; out output; Steady_state input; Fine_APEreq input; Coarse_completed input
function out = fcn( LOS, Steady_state, Fine_APEreq, Coarse_completed)

if Coarse_completed>0
    
        if sum(abs(LOS-Steady_state)-Fine_APEreq<0)==3
            out=1;
        else
            out=0;
        end
else 
        
    out=0;
    
end

== matlab function Simscape_Benchmark_SIM1/Checks on pointing requirements for initiating phase transitions /Check condition for a time window (C2F) ==
  data: u input; out output; sampling input; Transition_C2FtimeCheck input; Coarse_Completed input; Transition_C2FtimeCheck_reqNotMet input; out2 output
function [out,out2] = FUNZ(u, sampling, Transition_C2FtimeCheck,Coarse_Completed,Transition_C2FtimeCheck_reqNotMet)
persistent Counter_C2F fix_transitionC2F Counter_C2F_req_NotMet
% maybe an and to deactivate it completerly

out2=1; % I have to initialize it

if isempty(fix_transitionC2F)
    fix_transitionC2F=0;
end

if isempty(Counter_C2F) || u==0
    Counter_C2F=0;
elseif  u==1
    Counter_C2F=Counter_C2F+1;
end

% This second counter starts to count as soon as the slew is completed
if isempty(Counter_C2F_req_NotMet) || Coarse_Completed==0
    Counter_C2F_req_NotMet=0;
elseif  Coarse_Completed==1
    Counter_C2F_req_NotMet=Counter_C2F_req_NotMet+1;
end

Time_check=Counter_C2F*sampling;
Time_check_req_NotMet=Counter_C2F_req_NotMet*sampling;


if Time_check>=Transition_C2FtimeCheck
    out=1;
    fix_transitionC2F=1;
else
    out=0;
end

if fix_transitionC2F==1
     out=1;
     Time_check_req_NotMet=0;
     out2=1; % MEANS THAT THE REQUIREMENT IS MET
end

if Time_check_req_NotMet>=Transition_C2FtimeCheck_reqNotMet
    out=1;
    out2= 0;  % MEANS THAT THE REQUIREMENT IS not  MET
end
